simulink model "smart_manufacturing_robotics_cyber_physical_system_v2"  (R2012b)
settings: Solver=FixedStepDiscrete  StartTime=0.0  StopTime=34  RelTol=20e-5
model workspace (MAT data in the model file):
  ini_G_block_hpos = -0.4
  ini_G_block_vpos = 0.14
  block_height = 0.07
  ini_nozzle_pos = 0.3
  board_vpos = 0
  blockG = 2
  blockR = 1
  ini_R_block_vpos = 0.21
  ini_R_block_hpos = -0.4
  ini_B_block_vpos = 0.07
  ini_B_block_hpos = -0.4
  blockB = 3
  vpos_bottom = 0.07
  vpos_middle = 0.14
  vpos_top = 0.21
  order1_active = 'patch([0 1 1 0], [0.66 0.66 1 1], [0 0 1]);
patch([0 1 1 0], [0.33 0.33 0.66 0.66], [0 1 0]);
patch([0 1 1 0], [0 0 0.33 0.33], [1 0 0]);

color(''black'');
plot([0 1 1 0 0], [0 0 1 1 0]);
'
  order1_inactive = 'patch([0 1 1 0], [0.66 0.66 1 1], [0.5 0.5 1]);
patch([0 1 1 0], [0.33 0.33 0.66 0.66], [0.5 1 0.5]);
patch([0 1 1 0], [0 0 0.33 0.33], [1 0.5 0.5]);

color(''black'');
plot([0 1 1 0 0], [0 0 1 1 0]);
'
  order2_active = 'patch([0 1 1 0], [0.66 0.66 1 1], [0 1 0]);
patch([0 1 1 0], [0.33 0.33 0.66 0.66], [0 0 1]);
patch([0 1 1 0], [0 0 0.33 0.33], [1 0 0]);

color(''black'');
plot([0 1 1 0 0], [0 0 1 1 0]);
'
  order3_active = 'patch([0 1 1 0], [0.66 0.66 1 1], [0 1 0]);
patch([0 1 1 0], [0.33 0.33 0.66 0.66], [1 0 0]);
patch([0 1 1 0], [0 0 0.33 0.33], [0 0 1]);

color(''black'');
plot([0 1 1 0 0], [0 0 1 1 0]);
'
  order4_active = 'patch([0 1 1 0], [0.66 0.66 1 1], [0 0 1]);
patch([0 1 1 0], [0.33 0.33 0.66 0.66], [1 0 0]);
patch([0 1 1 0], [0 0 0.33 0.33], [0 1 0]);

color(''black'');
plot([0 1 1 0 0], [0 0 1 1 0]);
'
  order5_active = 'patch([0 1 1 0], [0.66 0.66 1 1], [1 0 0]);
patch([0 1 1 0], [0.33 0.33 0.66 0.66], [0 0 1]);
patch([0 1 1 0], [0 0 0.33 0.33], [0 1 0]);

color(''black'');
plot([0 1 1 0 0], [0 0 1 1 0]);
'
  order6_active = 'patch([0 1 1 0], [0.66 0.66 1 1], [1 0 0]);
patch([0 1 1 0], [0.33 0.33 0.66 0.66], [0 1 0]);
patch([0 1 1 0], [0 0 0.33 0.33], [0 0 1]);

color(''black'');
plot([0 1 1 0 0], [0 0 1 1 0]);
'
  order2_inactive = 'patch([0 1 1 0], [0.66 0.66 1 1], [0. 1 0.5]);
patch([0 1 1 0], [0.33 0.33 0.66 0.66], [0.5 0.5 1]);
patch([0 1 1 0], [0 0 0.33 0.33], [1 0.5 0.5]);

color(''black'');
plot([0 1 1 0 0], [0 0 1 1 0]);
'
  order3_inactive = 'patch([0 1 1 0], [0.66 0.66 1 1], [0.5 1 0.5]);
patch([0 1 1 0], [0.33 0.33 0.66 0.66], [1 0.5 0.5]);
patch([0 1 1 0], [0 0 0.33 0.33], [0.5 0.5 1]);

color(''black'');
plot([0 1 1 0 0], [0 0 1 1 0]);
'
  order4_inactive = 'patch([0 1 1 0], [0.66 0.66 1 1], [0.5 0.5 1]);
patch([0 1 1 0], [0.33 0.33 0.66 0.66], [1 0.5 0.5]);
patch([0 1 1 0], [0 0 0.33 0.33], [0.5 1 0.5]);

color(''black'');
plot([0 1 1 0 0], [0 0 1 1 0]);
'
  order5_inactive = 'patch([0 1 1 0], [0.66 0.66 1 1], [1 0.5 0.5]);
patch([0 1 1 0], [0.33 0.33 0.66 0.66], [0.5 0.5 1]);
patch([0 1 1 0], [0 0 0.33 0.33], [0.5 1 0.5]);

color(''black'');
plot([0 1 1 0 0], [0 0 1 1 0]);
'
  order6_inactive = 'patch([0 1 1 0], [0.66 0.66 1 1], [1 0.5 0.5]);
patch([0 1 1 0], [0.33 0.33 0.66 0.66], [0.5 1 0.5]);
patch([0 1 1 0], [0 0 0.33 0.33], [0.5 0.5 1]);

color(''black'');
plot([0 1 1 0 0], [0 0 1 1 0]);
'
settings Model: ExplicitPartitioning=on  Creator=pmosterm  LastModifiedBy=pmosterm
settings SolverCC: ZcThreshold=2e-5  MaxConsecutiveZCs=20  EnableConcurrentExecution=on  ConcurrentTasks=on  ZeroCrossAlgorithm=Adaptive  SolverResetMethod=Robust
settings DataIOCC: ExternalInput=take_snapshot,find_stack  LoadExternalInput=on  SignalLoggingSaveFormat=ModelDataLogs  SaveOutput=off  SignalLogging=off  DSMLogging=off  SaveTime=off
settings OptimizationCC: InlineParams=on
settings DebuggingCC: ReadBeforeWriteMsg=DisableAll  WriteAfterWriteMsg=DisableAll  WriteAfterReadMsg=DisableAll  AlgebraicLoopMsg=error  UnderspecifiedInitializationDetection=Simplified  FcnCallInpInsideContextMsg=EnableAllAsWarning  ModelReferenceExtraNoncontSigs=warning
settings GRTTargetCC: CombineOutputUpdateFcns=off  GRTInterface=on
settings ConfigurationSet: Description=SimMechanics 2G

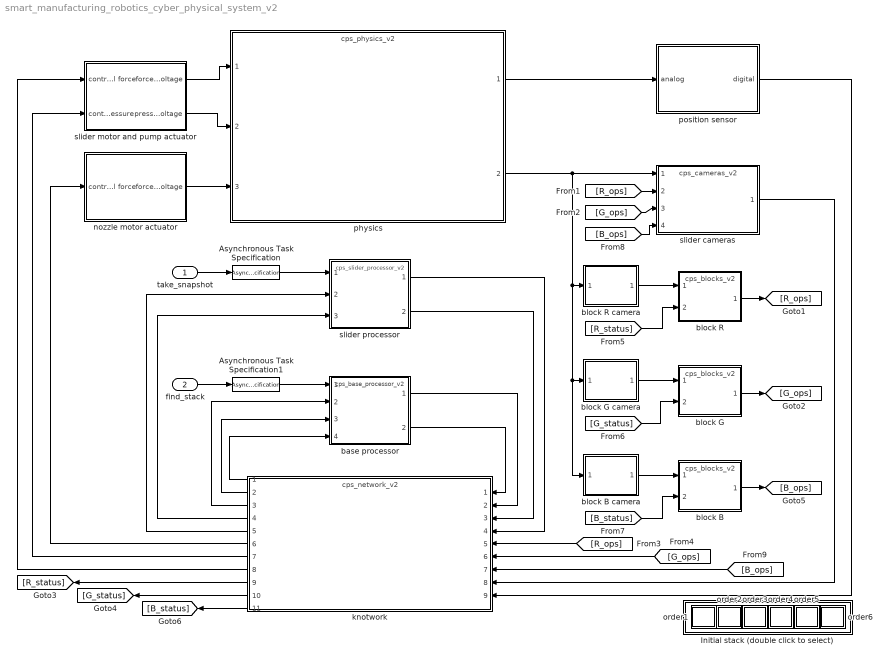
== system smart_manufacturing_robotics_cyber_physical_system_v2 ==
  take_snapshot : Inport  OutputFunctionCall=on
  find_stack : Inport  Port=2  OutputFunctionCall=on
  Asynchronous Task Specification : AsynchronousTaskSpecification  TaskPriority=5
  Asynchronous Task Specification1 : AsynchronousTaskSpecification
  Initial stack (double click to select) : Subsystem
      mask Display:
      | patch([0 1 1 0], [0 0 1 1], [0.8 0.8 0.8]);
      | plot([0 0 1 1 0], [0 1 1 0 0]);
  base processor : ModelReference  ModelNameDialog=cps_base_processor_v2  ParameterArgumentNames=board_vpos,block_height  ParameterArgumentValues=board_vpos, block_height  SimulationMode=Normal  ModelReferenceVersion=1.921  CopyOfModelName=cps_base_processor_v2  DefaultDataLogging=on
      mask Display: image(imread('images\processor_v12b_89x76.jpg'));
  block B : ModelReference  ModelNameDialog=cps_blocks_v2  ParameterArgumentNames=block  ParameterArgumentValues=blockB  SimulationMode=Normal  ModelReferenceVersion=1.769  CopyOfModelName=cps_blocks_v2  DefaultDataLogging=on
      mask Display: image(imread('images\processor_v12b_70x55.jpg'));
  block B camera : ModelReference  ModelNameDialog=cps_blockB_camera_v2  ParameterArgumentNames=ini_G_block_vpos,ini_B_block_vpos,block_height  ParameterArgumentValues=ini_G_block_vpos,ini_R_block_vpos,block_height  SimulationMode=Normal  ModelReferenceVersion=1.638  CopyOfModelName=cps_blockB_camera_v2  DefaultDataLogging=on
      mask Display: image(imread('images\block_with_camera_v27.jpg'));
  block G : ModelReference  ModelNameDialog=cps_blocks_v2  ParameterArgumentNames=block  ParameterArgumentValues=blockG  SimulationMode=Normal  ModelReferenceVersion=1.769  CopyOfModelName=cps_blocks_v2  DefaultDataLogging=on
      mask Display: image(imread('images\processor_v12b_70x55.jpg'));
  block G camera : ModelReference  ModelNameDialog=cps_blockG_camera_v2  ParameterArgumentNames=ini_G_block_vpos,ini_B_block_vpos,block_height  ParameterArgumentValues=ini_G_block_vpos,ini_R_block_vpos,block_height  SimulationMode=Normal  ModelReferenceVersion=1.621  CopyOfModelName=cps_blockG_camera_v2  DefaultDataLogging=on
      mask Display: image(imread('images\block_with_camera_v27a_60x44.jpg'));
  block R : ModelReference  ModelNameDialog=cps_blocks_v2  ParameterArgumentNames=block  ParameterArgumentValues=blockR  SimulationMode=Normal  ModelReferenceVersion=1.769  CopyOfModelName=cps_blocks_v2  DefaultDataLogging=on
      mask Display: image(imread('images\processor_v12b_70x55.jpg'));
  block R camera : ModelReference  ModelNameDialog=cps_blockR_camera_v2  ParameterArgumentNames=ini_G_block_vpos,ini_B_block_vpos,block_height  ParameterArgumentValues=ini_G_block_vpos,ini_R_block_vpos,block_height  SimulationMode=Normal  ModelReferenceVersion=1.630  CopyOfModelName=cps_blockR_camera_v2  DefaultDataLogging=on
      mask Display: image(imread('images\block_with_camera_v27b_60x44.jpg'));
  knotwork : ModelReference  ModelNameDialog=cps_network_v2  SimulationMode=Normal  ModelReferenceVersion=1.126  CopyOfModelName=cps_network_v2  DefaultDataLogging=on
      mask Display: image(imread('images\network_router_v98a_278x151.jpg'));
  nozzle motor actuator : Subsystem
      mask Display: image(imread('images\ncap_v35a_cut_115x76.jpg'));
  order1 : Subsystem
      settings: OpenFcn=|
      | temp = get_param(bdroot, 'modelworkspace');
      | temp.evalin('ini_B_block_vpos = vpos_top;');
      | temp.evalin('ini_G_block_vpos = vpos_middle;');
      | temp.evalin('ini_R_block_vpos = vpos_bottom;');
      | 
      | temp.evalin(order_callback);
      | 
      | clear temp;
      mask Display:
      | patch([0 1 1 0], [0.66 0.66 1 1], [0.5 0.5 1]);
      | patch([0 1 1 0], [0.33 0.33 0.66 0.66], [0.5 1 0.5]);
      | patch([0 1 1 0], [0 0 0.33 0.33], [1 0.5 0.5]);
      | 
      | color('black');
      | plot([0 1 1 0 0], [0 0 1 1 0]);
  order2 : Subsystem
      settings: OpenFcn=|
      | temp = get_param(bdroot, 'modelworkspace');
      | temp.evalin('ini_G_block_vpos = vpos_top;');
      | temp.evalin('ini_B_block_vpos = vpos_middle;');
      | temp.evalin('ini_R_block_vpos = vpos_bottom;');
      | 
      | temp.evalin(order_callback);
      | 
      | clear temp;
      mask Display:
      | patch([0 1 1 0], [0.66 0.66 1 1], [0. 1 0.5]);
      | patch([0 1 1 0], [0.33 0.33 0.66 0.66], [0.5 0.5 1]);
      | patch([0 1 1 0], [0 0 0.33 0.33], [1 0.5 0.5]);
      | 
      | color('black');
      | plot([0 1 1 0 0], [0 0 1 1 0]);
  order3 : Subsystem
      settings: OpenFcn=|
      | temp = get_param(bdroot, 'modelworkspace');
      | temp.evalin('ini_G_block_vpos = vpos_top;');
      | temp.evalin('ini_R_block_vpos = vpos_middle;');
      | temp.evalin('ini_B_block_vpos = vpos_bottom;');
      | 
      | temp.evalin(order_callback);
      | 
      | clear temp;
      mask Display:
      | patch([0 1 1 0], [0.66 0.66 1 1], [0.5 1 0.5]);
      | patch([0 1 1 0], [0.33 0.33 0.66 0.66], [1 0.5 0.5]);
      | patch([0 1 1 0], [0 0 0.33 0.33], [0.5 0.5 1]);
      | 
      | color('black');
      | plot([0 1 1 0 0], [0 0 1 1 0]);
  order4 : Subsystem
      settings: OpenFcn=|
      | temp = get_param(bdroot, 'modelworkspace');
      | temp.evalin('ini_B_block_vpos = vpos_top;');
      | temp.evalin('ini_R_block_vpos = vpos_middle;');
      | temp.evalin('ini_G_block_vpos = vpos_bottom;');
      | 
      | temp.evalin(order_callback);
      | 
      | clear temp;
      mask Display:
      | patch([0 1 1 0], [0.66 0.66 1 1], [0.5 0.5 1]);
      | patch([0 1 1 0], [0.33 0.33 0.66 0.66], [1 0.5 0.5]);
      | patch([0 1 1 0], [0 0 0.33 0.33], [0.5 1 0.5]);
      | 
      | color('black');
      | plot([0 1 1 0 0], [0 0 1 1 0]);
  order5 : Subsystem
      settings: OpenFcn=|
      | temp = get_param(bdroot, 'modelworkspace');
      | temp.evalin('ini_R_block_vpos = vpos_top;');
      | temp.evalin('ini_B_block_vpos = vpos_middle;');
      | temp.evalin('ini_G_block_vpos = vpos_bottom;');
      | 
      | temp.evalin(order_callback);
      | 
      | clear temp;
      mask Display:
      | patch([0 1 1 0], [0.66 0.66 1 1], [1 0.5 0.5]);
      | patch([0 1 1 0], [0.33 0.33 0.66 0.66], [0.5 0.5 1]);
      | patch([0 1 1 0], [0 0 0.33 0.33], [0.5 1 0.5]);
      | 
      | color('black');
      | plot([0 1 1 0 0], [0 0 1 1 0]);
  order6 : Subsystem
      settings: OpenFcn=|
      | temp = get_param(bdroot, 'modelworkspace');
      | temp.evalin('ini_R_block_vpos = vpos_top;');
      | temp.evalin('ini_G_block_vpos = vpos_middle;');
      | temp.evalin('ini_B_block_vpos = vpos_bottom;');
      | 
      | temp.evalin(order_callback);
      | 
      | clear temp;
      mask Display:
      | patch([0 1 1 0], [0.66 0.66 1 1], [1 0 0]);
      | patch([0 1 1 0], [0.33 0.33 0.66 0.66], [0 1 0]);
      | patch([0 1 1 0], [0 0 0.33 0.33], [0 0 1]);
      | 
      | color('black');
      | plot([0 1 1 0 0], [0 0 1 1 0]);
  physics : ModelReference  ModelNameDialog=cps_physics_v2  ParameterArgumentNames=ini_G_block_vpos,ini_G_block_hpos,ini_R_block_vpos,ini_R_block_hpos,ini_B_block_vpos,ini_B_block_hpos,ini_nozzle_pos,board_vpos,block_height  ParameterArgumentValues=ini_G_block_vpos, ini_G_block_hpos, ini_R_block_vpos, ini_R_block_hpos, ini_B_block_vpos, ini_B_block_hpos,ini_nozzle_pos, board_vpos, block_height  SimulationMode=Normal  ModelReferenceVersion=1.823  CopyOfModelName=cps_physics_v2  DefaultDataLogging=on
      mask Display: image(imread('images\smd_scene_v300a_316x218.jpg'));
  position sensor : Subsystem
      mask Display: image(imread('images\ncap_v35a_cut_115x76.jpg'));
  slider cameras : ModelReference  ModelNameDialog=cps_cameras_v2  ParameterArgumentNames=ini_G_block_vpos,ini_B_block_vpos,block_height  ParameterArgumentValues=ini_G_block_vpos,ini_R_block_vpos,block_height  SimulationMode=Normal  ModelReferenceVersion=1.655  CopyOfModelName=cps_cameras_v2  DefaultDataLogging=on
      mask Display: image(imread('images\smd_cams_v18a_115x76.jpg'));
  slider motor and pump actuator : Subsystem
      mask Display: image(imread('images\ncap_v35a_cut_115x76.jpg'));
  slider processor : ModelReference  ModelNameDialog=cps_slider_processor_v2  SimulationMode=Normal  ModelReferenceVersion=1.718  CopyOfModelName=cps_slider_processor_v2  DefaultDataLogging=on
      mask Display: image(imread('images\processor_v12b_89x76.jpg'));
  wires:
  knotwork/5 -> slider processor/2
  slider processor/1 -> knotwork/4
  slider processor/2 -> knotwork/3
  slider cameras/1 -> knotwork/8
  knotwork/2 -> base processor/3
  knotwork/6 -> nozzle motor actuator/1(control force)
  knotwork/7 -> slider motor and pump actuator/2(control pressure)
  knotwork/4 -> slider processor/3
  Asynchronous Task Specification/1 -> slider processor/1
  block R/1 -> [R_ops]
  block G/1 -> [G_ops]
  block G camera/1 -> block G/1
  block R camera/1 -> block R/1
  take_snapshot/1 -> Asynchronous Task Specification/1
  knotwork/3 -> base processor/2
  base processor/1 -> knotwork/2
  physics/2 -> slider cameras/1, block B camera/1, block G camera/1, block R camera/1
  knotwork/8 -> slider motor and pump actuator/1(control force)
  knotwork/1 -> base processor/4
  base processor/2 -> knotwork/1
  [R_ops] -> knotwork/5
  [G_ops] -> knotwork/6
  [G_status] -> block G/2
  [R_status] -> block R/2
  knotwork/10 -> [G_status]
  knotwork/9 -> [R_status]
  [R_ops] -> slider cameras/2
  [G_ops] -> slider cameras/3
  find_stack/1 -> Asynchronous Task Specification1/1
  Asynchronous Task Specification1/1 -> base processor/1
  slider motor and pump actuator/1(force voltage) -> physics/1
  slider motor and pump actuator/2(pressure voltage) -> physics/2
  nozzle motor actuator/1(force voltage) -> physics/3
  position sensor/1(digital) -> knotwork/9
  physics/1 -> position sensor/1(analog)
  block B/1 -> [B_ops]
  block B camera/1 -> block B/1
  [B_status] -> block B/2
  [B_ops] -> slider cameras/4
  [B_ops] -> knotwork/7
  knotwork/11 -> [B_status]

== system smart_manufacturing_robotics_cyber_physical_system_v2/Initial stack (double click to select) ==

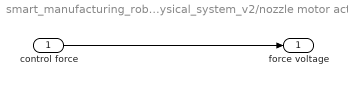
== system smart_manufacturing_robotics_cyber_physical_system_v2/nozzle motor actuator ==
  control force : Inport
  force voltage : Outport
  wires:
  control force/1 -> force voltage/1

== system smart_manufacturing_robotics_cyber_physical_system_v2/order1 ==

== system smart_manufacturing_robotics_cyber_physical_system_v2/order2 ==

== system smart_manufacturing_robotics_cyber_physical_system_v2/order3 ==

== system smart_manufacturing_robotics_cyber_physical_system_v2/order4 ==

== system smart_manufacturing_robotics_cyber_physical_system_v2/order5 ==

== system smart_manufacturing_robotics_cyber_physical_system_v2/order6 ==

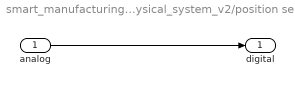
== system smart_manufacturing_robotics_cyber_physical_system_v2/position sensor ==
  analog : Inport
  digital : Outport
  wires:
  analog/1 -> digital/1

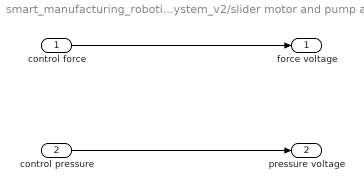
== system smart_manufacturing_robotics_cyber_physical_system_v2/slider motor and pump actuator ==
  control force : Inport
  control pressure : Inport  Port=2
  force voltage : Outport
  pressure voltage : Outport  Port=2
  wires:
  control force/1 -> force voltage/1
  control pressure/1 -> pressure voltage/1
